simulink model "pendulumSimB"  (R2018a)
settings: Solver=VariableStepAuto  StartTime=0.0  StopTime=100  MaxStep=0.001  RelTol=1e-3
InitFcn:
  | params
settings Model: Creator=mark  LastModifiedBy=mark

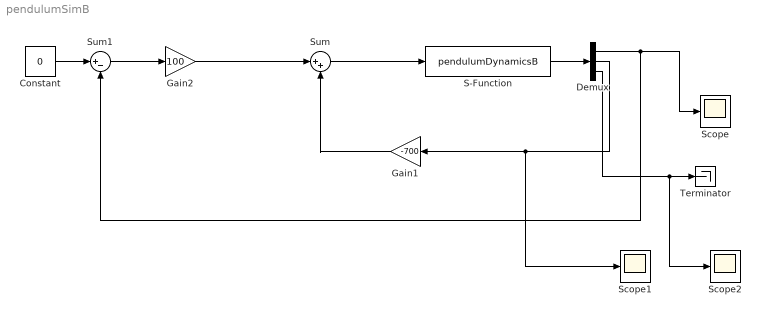
== system pendulumSimB ==
  Constant : Constant  Value=0
  Demux : Demux  Outputs=3
  Gain1 : Gain  Gain=-700
  Gain2 : Gain  Gain=100
  S-Function : S-Function  FunctionName=pendulumDynamicsB  Parameters=P  SFunctionDeploymentMode=off  EnableBusSupport=off
  Scope : Scope
  Scope1 : Scope
  Scope2 : Scope
  Sum : Sum  Inputs=|++
  Sum1 : Sum  Inputs=|+-
  Terminator : Terminator
  wires:
  S-Function/1 -> Demux/1
  Demux/1 -> Sum1/2, Scope/1
  Sum1/1 -> Gain2/1
  Gain2/1 -> Sum/1
  Constant/1 -> Sum1/1
  Sum/1 -> S-Function/1
  Demux/2 -> Scope1/1, Gain1/1
  Gain1/1 -> Sum/2
  Demux/3 -> Scope2/1, Terminator/1
